simulink model "HITL_Unreal_Visualization"  (R2026a)
settings: Solver=VariableStepAuto  StopTime=inf
undefined symbols (not defined in the file): f
libraries: uavmavlinklib x3, uavsim3dlib x2, sim3dlib x1, instrumentlib x1
settings Model: Creator=The MathWorks, Inc.  LastModifiedBy=The MathWorks, Inc.

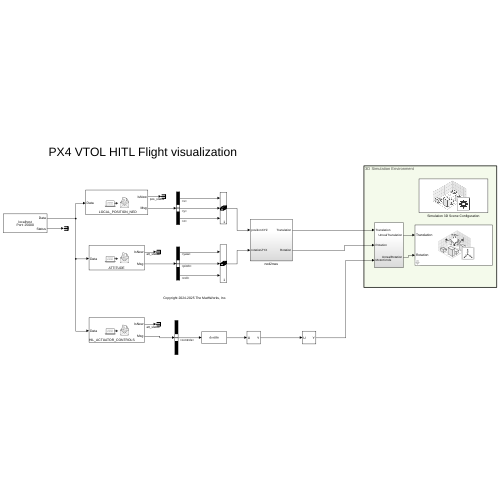
[thumbnail: Simulink's stored preview of the top-level diagram]
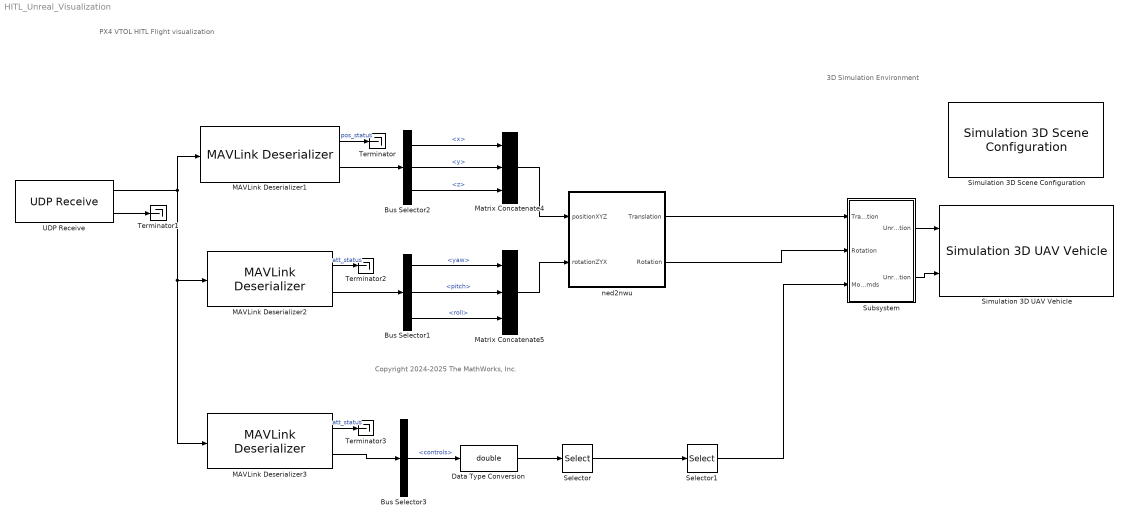
== system HITL_Unreal_Visualization ==
  note: 3D Simulation Environment
  note: Copyright 2024-2025 The MathWorks, Inc.
  note: PX4 VTOL HITL Flight visualization
  Bus Selector1 : BusSelector  OutputSignals=Payload.yaw,Payload.pitch,Payload.roll
  Bus Selector2 : BusSelector  OutputSignals=Payload.x,Payload.y,Payload.z
  Bus Selector3 : BusSelector  OutputSignals=Payload.controls
  Data Type Conversion : DataTypeConversion  OutDataTypeStr=double  SaturateOnIntegerOverflow=off  RndMeth=Floor
  MAVLink Deserializer1 : uavmavlinklib/MAVLink Deserializer  dialectSource=Select from standard MAVLink dialects  dialect=common.xml  dialectCustom=D:\px4_110\Firmware\mavlink\include\mavlink\v2.0\message_definitions\common.xml  version=2  messageType=LOCAL_POSITION_NED  inputDataLength=off  SystemIDFilter=off  systemID=1  ComponentIDFilter=off  componentID=1  queueMsg=off  queueMsgSize=50  dropNum=off
  MAVLink Deserializer2 : uavmavlinklib/MAVLink Deserializer  dialectSource=Select from standard MAVLink dialects  dialect=common.xml  dialectCustom=D:\px4_110\Firmware\mavlink\include\mavlink\v2.0\message_definitions\common.xml  version=2  messageType=ATTITUDE  inputDataLength=off  SystemIDFilter=off  systemID=1  ComponentIDFilter=off  componentID=1  queueMsg=off  queueMsgSize=50  dropNum=off
  MAVLink Deserializer3 : uavmavlinklib/MAVLink Deserializer  dialectSource=Select from standard MAVLink dialects  dialect=common.xml  dialectCustom=D:\px4_110\Firmware\mavlink\include\mavlink\v2.0\message_definitions\common.xml  version=2  messageType=HIL_ACTUATOR_CONTROLS  inputDataLength=off  SystemIDFilter=off  systemID=1  ComponentIDFilter=off  componentID=1  queueMsg=off  queueMsgSize=50  dropNum=off
  Matrix Concatenate4 : Concatenate  NumInputs=3  Mode=Multidimensional array
  Matrix Concatenate5 : Concatenate  NumInputs=3  Mode=Multidimensional array
  Selector : Selector  InputPortWidth=16  IndexOptions=Index vector (dialog)  Indices=[1:9]  OutputSizes=1
  Selector1 : Selector  InputPortWidth=9  IndexOptions=Index vector (dialog)  Indices=[1:6]  OutputSizes=1
  Simulation 3D Scene Configuration : sim3dlib/Simulation 3D Scene Configuration  Priority=0  ProjectFormat=Unreal Editor  SceneDesc=US city block  ProjectName=Y:\37\mpadhiya.Buav.j2460529.1\matlab\toolbox\shared\sim3d_projects\automotive_project_windows\UE\WindowsNoEditor\VehicleSimulation.exe  ScenePath=/Game/Maps/USCityBlock  UEProjPath=D:\AutoVrtlEnv\AutoVrtlEnv.uproject  EnableOpenDRIVE=off  vehTagList={'Custom';'Scene Origin';'VTOL_Vehicle'}  vehTag=VTOL_Vehicle  AttachedCameraRelativeTranslation=[0 0 0]  FreeCameraDefaultInitialTranslation=[-6, 0, 2]  AttachedCameraRelativeRotation=[0 0 0]  FreeCameraDefaultInitialRotation=[0, -15, 0]  ViewpointName=Custom  FreeCameraInitialTranslation=[0, 0, 0]  FreeCameraInitialRotation=[0, 0, 0]  OpVisEn=off  Ts=1/10  EnableWindow=on  EnableRemoteAccess=off  SimulationMode=CoSimulation  SimulateUsing=Interpreted execution  EnableAnimationRecording=off  OverrideDefaultRecording=off  AnimationRecordingFileName=sim3dAnimation.mat  AnimationRecordingInterval=[0 inf]  EnableWeather=off  SunAzimuth=90  SunAltitude=40.0  EnableGeospatialSun=off  Latitude=0  Longitude=0  Date=2023-01-01  Time=10:30:00  GeoTimeZone=-5.0  SunDaylightSaving=off  wind=1  clouds=10  EnableVolumetricClouds=off  CloudCoverage=0  CloudAltitude=6  fog=0  rain=0  RaindropsEffect=off  SnowDensity=0  EnableGeospatial=off  TilesetSource=Earth terrain  UseTrueOrigin=off  OriginHeight=200  OriginLatitude=40.744652  OriginLongitude=-73.988864  MapStyle=Aerial  AdditionalAssetIDs=[]  UseAdvancedSunSky=off  SolarTime=11  TimeZone=-5  Day=21  Month=9  Year=2022  UseDaylightSavingTime=on  DSTStartDay=10  DSTStartMonth=3  DSTEndDay=3  DSTEndMonth=11  DSTSwitchHour=2  sensorTag=MainCamera1  sensorId=1  sensorName=MainCamera1  mountLoc=Origin  offsetFlag=off  tmountOffset=[0, 0, 0]  rmountOffset=[0, 0, 0]  HorizontalResolution=1280  VerticalResolution=720  HorizontalFOV=60  mountPoint=[0 0 0]  mountOrientation=[0 0 0]  aMode=4  ID=1  GeoTrigger=Inactive  ViewNameList={'Custom'}  ViewTranslationList={'[0 0 0]'}  ViewRotationList={'[0 0 0]'}
      settings: LibrarySourceBlock=uavsim3dlib/Simulation 3D Scene Configuration
  Simulation 3D UAV Vehicle : uavsim3dlib/Simulation 3D UAV Vehicle  Priority=-1  Mesh=Custom  MeshPath=SkeletalMesh'/Game/EVTOL/VTOLAsset.VTOLAsset'  Color=Black  ActorName=VTOL_Vehicle  UseGlobalFrame=off  InitialTranslation=[0 0 0]  InitialRotation=[0 0 0]  InitialTranslationGlobal=[0 0 0]  InitialGeoOrigin=[0 0 0]  InitialRotationGlobal=[0 0 0]  SampleTime=0.1  ActorType=SimulinkVehicle  ID=C  aMode=4  ActorTag=VTOL_Vehicle
  Subsystem : Subsystem
  Terminator{,1..3} (4 alike) : Terminator
  UDP Receive : instrumentlib/UDP Receive  LocalAddress=localhost  LocalPort=25000  EnablePortSharing=off  Host=localhost  Port=9090  GetLatestData=on  DataSize="[1  512]"  DataType=uint8  ASCIIFormatting=%f,  Terminator=LF  CustomTerminator=10  ByteOrder=big-endian  EnableBlockingMode=off  Timeout=10  SampleTime=0.01  SimulateUsing=Interpreted execution
  ned2nwu : Subsystem
  wires:
  MAVLink Deserializer1/2 -> Bus Selector2/1
  MAVLink Deserializer1/1 -> Terminator/1  "pos_status"
  ned2nwu/1(Translation) -> Subsystem/1(Translation)
  Bus Selector2/1 -> Matrix Concatenate4/1  "<x>"
  Subsystem/2(UnrealRotation) -> Simulation 3D UAV Vehicle/2
  UDP Receive/2 -> Terminator1/1
  UDP Receive/1 -> MAVLink Deserializer3/1, MAVLink Deserializer2/1, MAVLink Deserializer1/1
  Bus Selector2/3 -> Matrix Concatenate4/3  "<z>"
  MAVLink Deserializer2/2 -> Bus Selector1/1
  MAVLink Deserializer2/1 -> Terminator2/1  "att_status"
  Bus Selector1/1 -> Matrix Concatenate5/1  "<yaw>"
  Subsystem/1(UnrealTranslation) -> Simulation 3D UAV Vehicle/1
  Bus Selector1/2 -> Matrix Concatenate5/2  "<pitch>"
  Matrix Concatenate5/1 -> ned2nwu/2(rotationZYX)
  Bus Selector2/2 -> Matrix Concatenate4/2  "<y>"
  Matrix Concatenate4/1 -> ned2nwu/1(positionXYZ)
  Bus Selector1/3 -> Matrix Concatenate5/3  "<roll>"
  MAVLink Deserializer3/1 -> Terminator3/1  "att_status"
  MAVLink Deserializer3/2 -> Bus Selector3/1
  Data Type Conversion/1 -> Selector/1
  Selector/1 -> Selector1/1
  Bus Selector3/1 -> Data Type Conversion/1  "<controls>"
  ned2nwu/2(Rotation) -> Subsystem/2(Rotation)
  Selector1/1 -> Subsystem/3(MotorCmds)

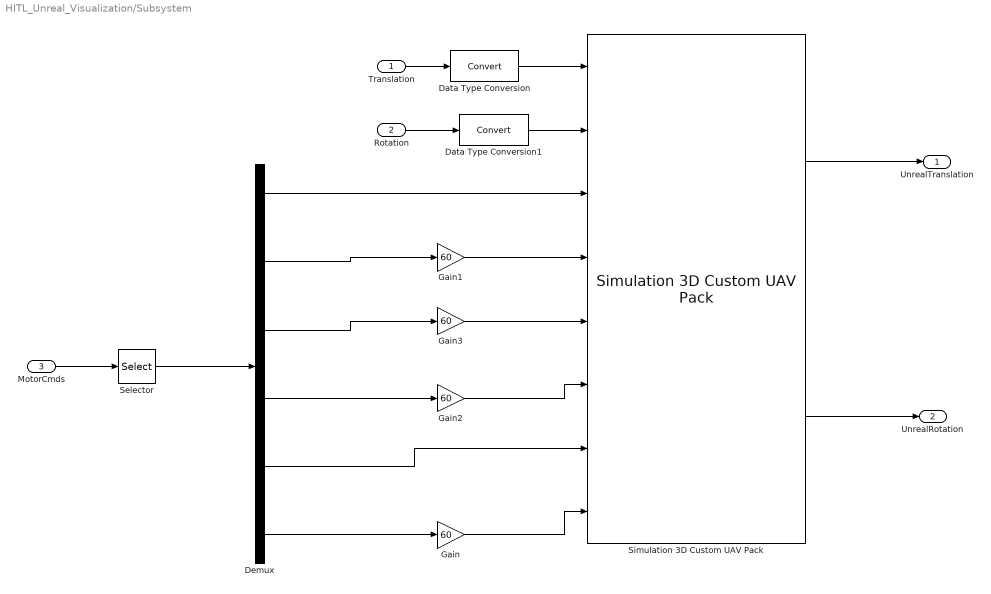
== system HITL_Unreal_Visualization/Subsystem ==
  Translation : Inport
  Rotation : Inport  Port=2
  MotorCmds : Inport  Port=3
  Data Type Conversion : DataTypeConversion  SaturateOnIntegerOverflow=off  RndMeth=Floor
  Data Type Conversion1 : DataTypeConversion  SaturateOnIntegerOverflow=off  RndMeth=Floor
  Demux : Demux  Outputs=6
  Gain{,1..3} (4 alike) : Gain  Gain=60
  Selector : Selector  InputPortWidth=6  IndexOptions=Index vector (dialog)  Indices=[5 1 4 3 6 2]  OutputSizes=1
  Simulation 3D Custom UAV Pack : uavsim3dlib/Simulation 3D Custom UAV Pack  enableMotor1Tilt=on  enableMotor2Tilt=off  enableMotor3Tilt=off  enableMotor4Tilt=on  enableMotor5Tilt=off  enableMotor6Tilt=off  enableMotor7Tilt=off  enableMotor8Tilt=off  enableRotor1RPM=on  enableRotor2RPM=on  enableRotor3RPM=on  enableRotor4RPM=on  enableRotor5RPM=off  enableRotor6RPM=off  enableRotor7RPM=off  enableRotor8RPM=off
  UnrealTranslation : Outport
  UnrealRotation : Outport  Port=2
  wires:
  Demux/6 -> Gain/1
  Simulation 3D Custom UAV Pack/1 -> UnrealTranslation/1
  Gain2/1 -> Simulation 3D Custom UAV Pack/6
  Demux/2 -> Gain1/1
  Demux/4 -> Gain2/1
  Simulation 3D Custom UAV Pack/2 -> UnrealRotation/1
  Gain1/1 -> Simulation 3D Custom UAV Pack/4
  Translation/1 -> Data Type Conversion/1
  Demux/3 -> Gain3/1
  Gain/1 -> Simulation 3D Custom UAV Pack/8
  Rotation/1 -> Data Type Conversion1/1
  Demux/5 -> Simulation 3D Custom UAV Pack/7
  Gain3/1 -> Simulation 3D Custom UAV Pack/5
  Demux/1 -> Simulation 3D Custom UAV Pack/3
  MotorCmds/1 -> Selector/1
  Selector/1 -> Demux/1
  Data Type Conversion/1 -> Simulation 3D Custom UAV Pack/1
  Data Type Conversion1/1 -> Simulation 3D Custom UAV Pack/2

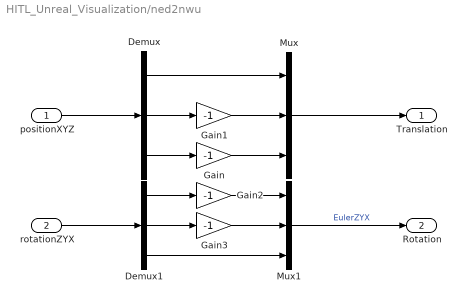
== system HITL_Unreal_Visualization/ned2nwu ==
  positionXYZ : Inport
  rotationZYX : Inport  Port=2
  Demux : Demux  Outputs=3
  Demux1 : Demux  Outputs=3
  Gain{,1..3} (4 alike) : Gain  Gain=-1
  Mux : Mux  Inputs=3
  Mux1 : Mux  Inputs=3
  Translation : Outport
  Rotation : Outport  Port=2
  wires:
  Mux/1 -> Translation/1
  Mux1/1 -> Rotation/1  "EulerZYX"
  Demux1/1 -> Gain2/1
  Demux1/2 -> Gain3/1
  Demux1/3 -> Mux1/3
  Demux/3 -> Gain/1
  Demux/2 -> Gain1/1
  Demux/1 -> Mux/1
  Gain/1 -> Mux/3
  Gain1/1 -> Mux/2
  Gain3/1 -> Mux1/2
  Gain2/1 -> Mux1/1
  positionXYZ/1 -> Demux/1
  rotationZYX/1 -> Demux1/1
